simulink model "Cont"  (R2021a)
settings: Solver=ode45  StartTime=0.0  StopTime=5  RelTol=1e-9
undefined symbols (not defined in the file or in its folder): Kp_tuned
settings Model: Creator=domin  LastModifiedBy=domin
settings SolverCC: ZeroCrossAlgorithm=Adaptive  AlgebraicLoopSolver=TrustRegion
settings DebuggingCC: IgnoredZcDiagnostic=none  SFMachineParentedDataDiag=warning

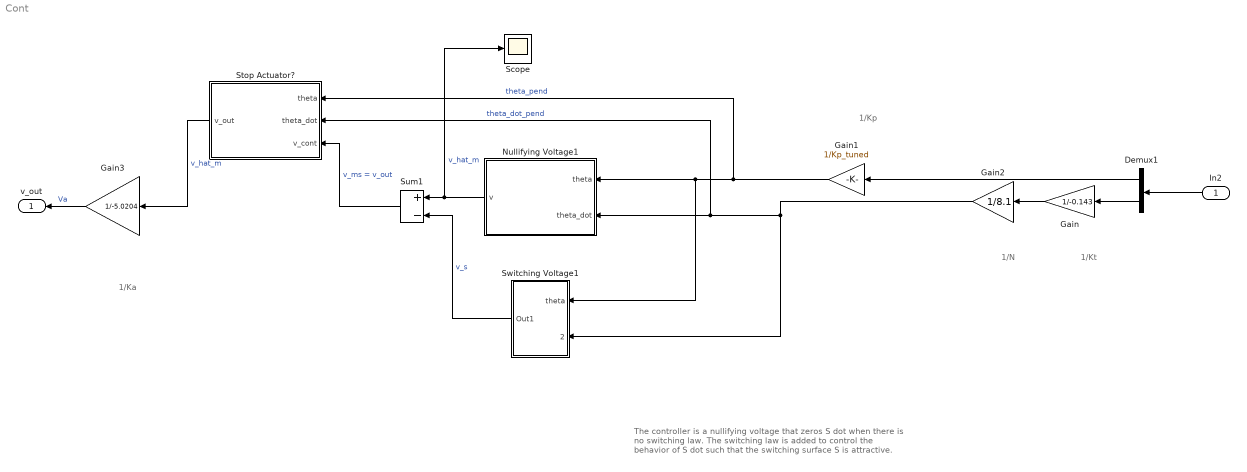
== system Cont ==
  note: 1/Ka
  note: 1/Kt
  note: 1/N
  note: 1/Kp
  note: The controller is a nullifying voltage that zeros S dot
      | when there is no switching law. The switching law is added
      | to control the behavior of S dot such that the switching surface
      | S is attractive.
  In2 : Inport  SampleTime=.01
  Demux1 : Demux  Outputs=2
  Gain : Gain  Gain=1/-0.143
  Gain1 : Gain  Gain=1/Kp_tuned
  Gain2 : Gain  Gain=1/8.1
  Gain3 : Gain  Gain=1/-5.0204
  Nullifying Voltage1 : MATLAB Function  TreatAsAtomicUnit=on
  Scope : Scope
  Stop Actuator? : MATLAB Function  TreatAsAtomicUnit=on
  Sum1 : Sum  Inputs=+-
  Switching Voltage1 : Subsystem
  v_out : Outport
  wires:
  Stop Actuator?/1(v_out) -> Gain3/1  "v_hat_m"
  Sum1/1 -> Stop Actuator?/3(v_cont)  "v_ms = v_out"
  Demux1/1 -> Gain1/1
  Demux1/2 -> Gain/1
  Nullifying Voltage1/1(v) -> Scope/1, Sum1/1  "v_hat_m"
  Switching Voltage1/1(Out1) -> Sum1/2  "v_s"
  In2/1 -> Demux1/1
  Gain/1 -> Gain2/1
  Gain2/1 -> Switching Voltage1/2(theta_dot), Stop Actuator?/2(theta_dot), Nullifying Voltage1/2(theta_dot)  "theta_dot_pend"
  Gain1/1 -> Stop Actuator?/1(theta), Nullifying Voltage1/1(theta), Switching Voltage1/1(theta)  "theta_pend"
  Gain3/1 -> v_out/1  "Va"

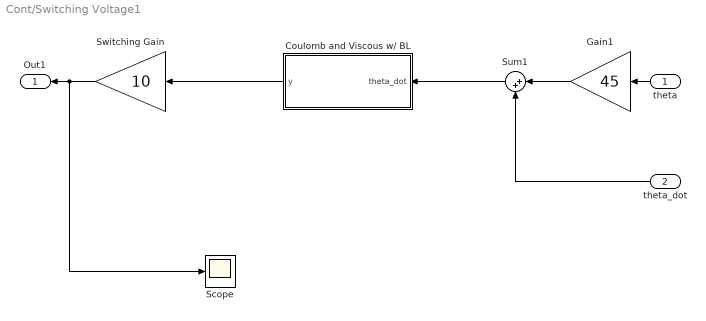
== system Cont/Switching Voltage1 ==
  theta : Inport
  theta_dot : Inport  Port=2
  Coulomb and Viscous w/ BL : MATLAB Function  TreatAsAtomicUnit=on
  Gain1 : Gain  Gain=45
  Scope : Scope
  Sum1 : Sum  Inputs=|++
  Switching Gain : Gain  Gain=10
  Out1 : Outport
  wires:
  Gain1/1 -> Sum1/1
  theta/1 -> Gain1/1
  Switching Gain/1 -> Scope/1, Out1/1
  Sum1/1 -> Coulomb and Viscous w/ BL/1(theta_dot)
  theta_dot/1 -> Sum1/2
  Coulomb and Viscous w/ BL/1(y) -> Switching Gain/1

== matlab function Cont/Nullifying Voltage1 ==
  data: theta input; theta_dot input; v output
function v = fcn(theta, theta_dot)

lambda_n = 45;
v = 0.3501*theta_dot - 1.0684*sign(theta_dot) - 0.6600*sin(theta_dot)...
    - 0.1144*lambda_n*theta_dot;

== matlab function Cont/Stop Actuator? ==
  data: theta input; theta_dot input; v_out output; v_cont input
function v_out = fcn(theta, theta_dot, v_cont)

if norm([theta theta_dot])<=.3
    
    v_out = 0;
    
else
    
    v_out = v_cont;
end

== matlab function Cont/Switching Voltage1/Coulomb and Viscous w// BL ==
  data: theta_dot input; y output
function y = fcn(theta_dot)

y = erf(1.25*theta_dot);
